simulink model "Project_2"  (R2024a)
settings: Solver=VariableStepAuto  StartTime=0.0  StopTime=10.0  RelTol=1e-3
values from neighbouring files (symbols this model uses):
  A = 2    [Project_2Mscript.m]
  F = 1    [Project3Mscript.m]    (also in Project4Mscript.m; Project7Mscript.m; Project_2Mscript.m = 5)
  Ti = 3    [Project_2Mscript.m]
libraries: simulink x1
settings Model: Creator=harsh  LastModifiedBy=harsh

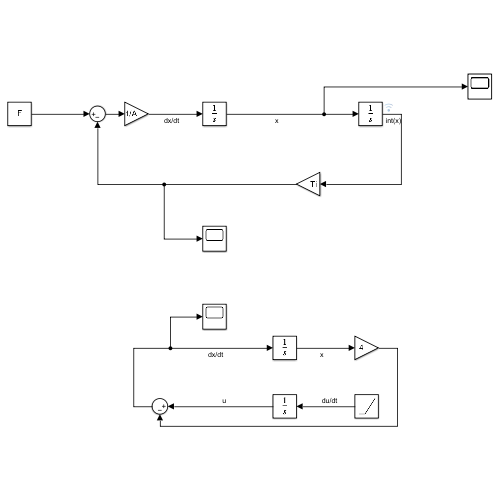
[thumbnail: Simulink's stored preview of the top-level diagram]
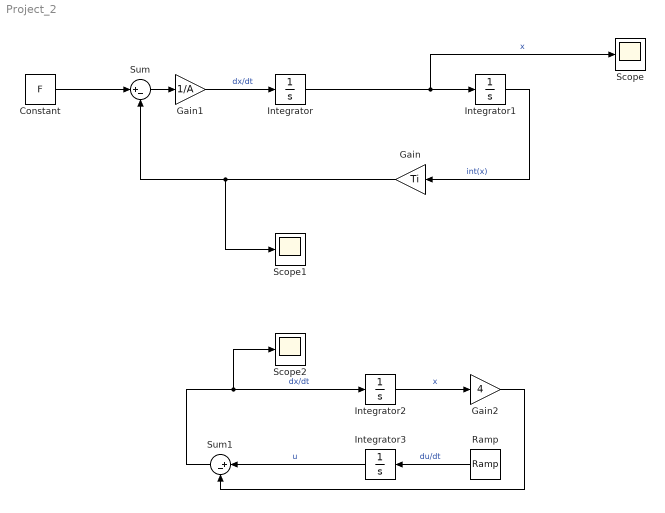
== system Project_2 ==
  Constant : Constant  Value=F
  Gain : Gain  Gain=Ti
  Gain1 : Gain  Gain=1/A
  Gain2 : Gain  Gain=4
  Integrator{,1..3} (4 alike) : Integrator
  Ramp : simulink/Sources/Ramp  slope=1  start=0  InitialOutput=0
  Scope : Scope
  Scope1 : Scope
  Scope2 : Scope
  Sum : Sum  Inputs=|+-
  Sum1 : Sum  Inputs=|+-
  wires:
  Constant/1 -> Sum/1
  Gain1/1 -> Integrator/1  "dx/dt"
  Integrator/1 -> Scope/1, Integrator1/1  "x"
  Integrator1/1 -> Gain/1  "int(x)"
  Gain/1 -> Scope1/1, Sum/2
  Sum/1 -> Gain1/1
  Sum1/1 -> Scope2/1, Integrator2/1  "dx/dt"
  Integrator2/1 -> Gain2/1  "x"
  Gain2/1 -> Sum1/2
  Ramp/1 -> Integrator3/1  "du/dt"
  Integrator3/1 -> Sum1/1  "u"
